simulink model "output_opt_lookup_formation_sim2"  (R2017b)
settings: Solver=VariableStepAuto  StartTime=0.0  StopTime=runtime  RelTol=1e-3
values from neighbouring files (symbols this model uses):
  ess_init_soc = 0.6    [ev_sim_init2.m]
  input_motor_speed = mtr_speed_rad(j)    [output_opt_lookup_formation2.m]
  input_motor_torque = mtr_torque_Nm(i)    [output_opt_lookup_formation2.m]
  K_high = 2    [ev_sim_init2.m]
  K_low = 1    [ev_sim_init2.m]
  TA = torque_allocation(k)    [output_opt_lookup_formation2.m]
undefined symbols (not defined in the file or in its folder): A_frontal, ap00, ap01, ap02, ap03, ap10, ap11, ap12, ap20, ap21, ap30, C_d, ess_cap_scale, ess_fixtemp, ess_max_ah_cap, ess_max_volts, ess_min_volts, ess_module_num, ess_r_chg, ess_r_dis, ess_res_scale_coef, ess_res_scale_fun, ess_soc, ess_tmp, ess_voc, f_rolling, FR, g_gravity, m_map_spd, m_max_trq_IM, m_max_trq_SR, m_min_volts, M_total, p00, p01, p02, p03, p10, p11, p12, p20, p21, p30, R_tire, rho_air
libraries: simulink x3
settings Model: Creator=Robert Wygant  LastModifiedBy=Robert Wygant
settings SolverCC: ZeroCrossControl=DisableAll
settings DebuggingCC: MaxConsecutiveZCsMsg=none

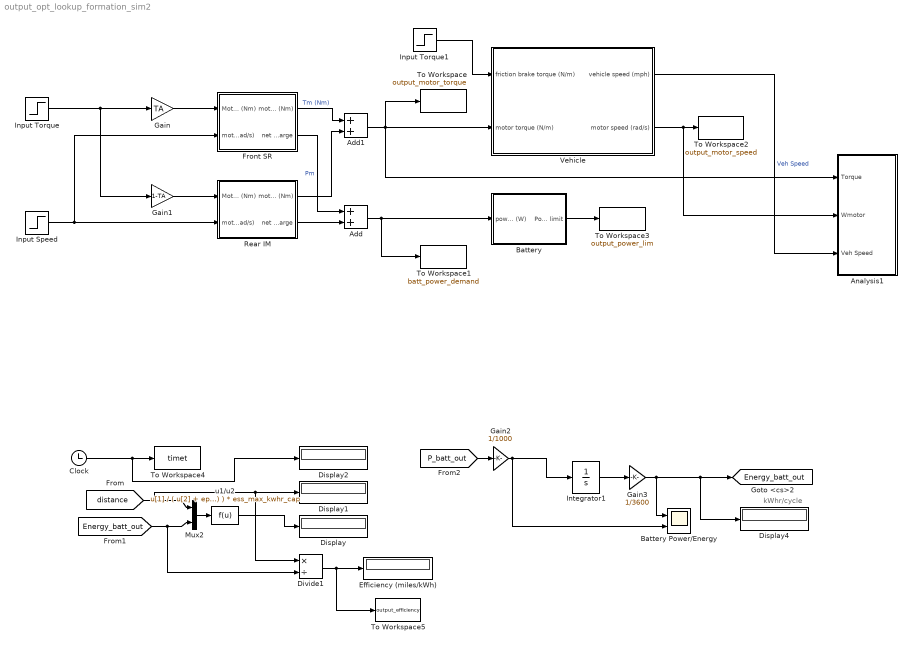
== system output_opt_lookup_formation_sim2 ==
  note: kWhr/cycle
  Add : Sum
  Add1 : Sum
  Analysis1 : Subsystem
  Battery : Subsystem
      mask Display: disp('Battery')
  Battery Power/Energy : Scope  NumInputPorts=2
      settings: Description=Power/Energy
  Clock : Clock
  Display{,1..2,4} (4 alike) : Display
  Divide1 : Product  Inputs=*/
  Efficiency (miles/kWh) : Display
  Front SR : Subsystem
      mask Display: disp('Electric\nMotor')
  Gain : Gain  Gain=TA
  Gain1 : Gain  Gain=1-TA
  Gain2 : Gain  Gain=1/1000  SaturateOnIntegerOverflow=on  OutDataTypeStr=Inherit: Same as input  ParamDataTypeStr=Inherit: Same as input
  Gain3 : Gain  Gain=1/3600  SaturateOnIntegerOverflow=on  OutDataTypeStr=Inherit: Same as input  ParamDataTypeStr=Inherit: Same as input
  Input Speed : Step  Time=0  After=input_motor_speed  SampleTime=0
  Input Torque : Step  Time=0  After=input_motor_torque  SampleTime=0
  Input Torque1 : Step  Time=0.01  After=0  SampleTime=0
  Integrator1 : Integrator  LowerSaturationLimit=0
  Mux2 : Mux  Inputs=2
  Rear IM : Subsystem
      mask Display: disp('Electric\nMotor')
  To Workspace : ToWorkspace  VariableName=output_motor_torque  SampleTime=-1
      settings: Save2DSignal=2-D array (concatenate along first dimension)
  To Workspace1 : ToWorkspace  VariableName=batt_power_demand  SaveFormat=Structure  SampleTime=-1
      settings: Save2DSignal=2-D array (concatenate along first dimension)
  To Workspace2 : ToWorkspace  VariableName=output_motor_speed  SampleTime=-1
      settings: Save2DSignal=2-D array (concatenate along first dimension)
  To Workspace3 : ToWorkspace  VariableName=output_power_lim  SampleTime=-1
      settings: Save2DSignal=2-D array (concatenate along first dimension)
  To Workspace4 : ToWorkspace  VariableName=timet  SampleTime=-1
  To Workspace5 : ToWorkspace  VariableName=output_efficiency  SampleTime=-1
      settings: Save2DSignal=2-D array (concatenate along first dimension)
  Vehicle : Subsystem
      mask Display: disp('Vehicle \nDynamic Model')
  u1/u2 : Fcn  Expr=u[1] / ( u[2] + eps*(u[2] == 0) ) * ess_max_kwhr_cap
  tag scope: Energy_batt_out=global
  wires:
  Front SR/1(motor torque output (Nm)) -> Add1/1  "Tm (Nm)"
  Rear IM/1(motor torque output (Nm)) -> Add1/2
  Add/1 -> Battery/1(power req'd into bus (W)), To Workspace1/1
  Front SR/2(net Power >0 discharge <0 charge) -> Add/1  "Pm"
  Rear IM/2(net Power >0 discharge <0 charge) -> Add/2
  Gain/1 -> Front SR/1(Motor demand Torque (Nm))
  Gain1/1 -> Rear IM/1(Motor demand Torque (Nm))
  Input Torque/1 -> Gain1/1, Gain/1
  Input Speed/1 -> Rear IM/2(motor speed (rad/s)), Front SR/2(motor speed (rad/s))
  Vehicle/1(vehicle speed (mph)) -> Analysis1/3(Veh Speed)  "Veh Speed"
  Add1/1 -> Vehicle/2(motor torque (N/m)), Analysis1/1(Torque), To Workspace/1
  Input Torque1/1 -> Vehicle/1(friction brake torque (N/m))
  Vehicle/2(motor speed (rad/s)) -> Analysis1/2(Wmotor), To Workspace2/1
  Divide1/1 -> To Workspace5/1, Efficiency (miles/kWh)/1
  Gain3/1 -> [Energy_batt_out], Display4/1, Battery Power/Energy/1
  Clock/1 -> To Workspace4/1, Display2/1
  [P_batt_out] -> Gain2/1
  [Energy_batt_out] -> Divide1/2, Mux2/2
  Gain2/1 -> Integrator1/1, Battery Power/Energy/2
  Mux2/1 -> u1/u2/1
  [distance] -> Divide1/1, Display1/1, Mux2/1
  u1/u2/1 -> Display/1
  Integrator1/1 -> Gain3/1
  Battery/1(Power limit) -> To Workspace3/1

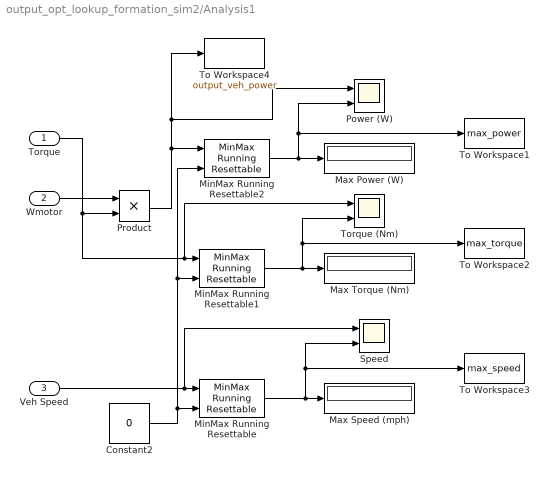
== system output_opt_lookup_formation_sim2/Analysis1 ==
  Torque : Inport
  Wmotor : Inport  Port=2
  Veh Speed : Inport  Port=3
  Constant2 : Constant  Value=0  VectorParams1D=off  SampleTime=-1
  Max Power (W) : Display
  Max Speed (mph) : Display
  Max Torque (Nm) : Display
  MinMax Running Resettable : simulink/Math Operations/MinMax Running Resettable  Function=max  vinit=0.0
  MinMax Running Resettable1 : simulink/Math Operations/MinMax Running Resettable  Function=max  vinit=0.0
  MinMax Running Resettable2 : simulink/Math Operations/MinMax Running Resettable  Function=max  vinit=0.0
  Power (W) : Scope  NumInputPorts=2
  Product : Product
  Speed : Scope  NumInputPorts=2
  To Workspace1 : ToWorkspace  VariableName=max_power  SampleTime=-1
      settings: Save2DSignal=2-D array (concatenate along first dimension)
  To Workspace2 : ToWorkspace  VariableName=max_torque  SampleTime=-1
      settings: Save2DSignal=2-D array (concatenate along first dimension)
  To Workspace3 : ToWorkspace  VariableName=max_speed  SampleTime=-1
      settings: Save2DSignal=2-D array (concatenate along first dimension)
  To Workspace4 : ToWorkspace  VariableName=output_veh_power  SampleTime=-1
      settings: Save2DSignal=2-D array (concatenate along first dimension)
  Torque (Nm) : Scope  NumInputPorts=2
  wires:
  Veh Speed/1 -> Speed/1, MinMax Running Resettable/1
  Wmotor/1 -> Product/1
  Torque/1 -> Torque (Nm)/1, MinMax Running Resettable1/1, Product/2
  Product/1 -> MinMax Running Resettable2/1, To Workspace4/1, Power (W)/1
  Constant2/1 -> MinMax Running Resettable2/2, MinMax Running Resettable1/2, MinMax Running Resettable/2
  MinMax Running Resettable1/1 -> To Workspace2/1, Torque (Nm)/2, Max Torque (Nm)/1
  MinMax Running Resettable/1 -> To Workspace3/1, Speed/2, Max Speed (mph)/1
  MinMax Running Resettable2/1 -> To Workspace1/1, Power (W)/2, Max Power (W)/1

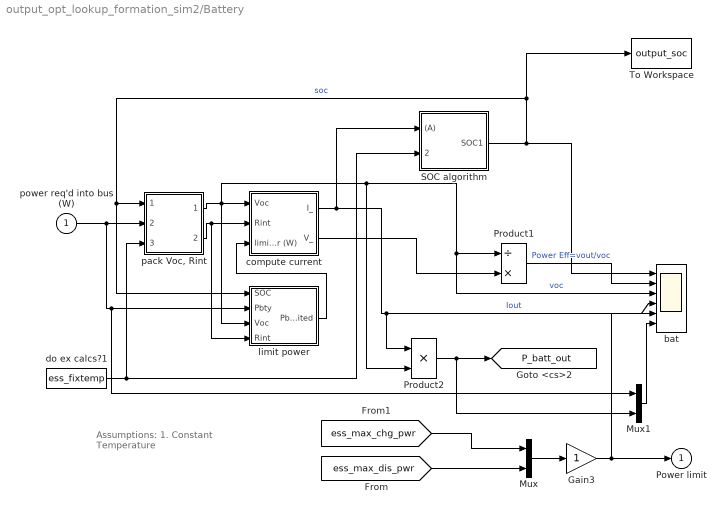
== system output_opt_lookup_formation_sim2/Battery ==
  note: Assumptions:
      | 1. Constant Temperature
  power req'd into bus (W) : Inport
  Gain3 : Gain  SaturateOnIntegerOverflow=on  OutDataTypeStr=Inherit: Same as input  ParamDataTypeStr=Inherit: Same as input
  Mux : Mux  Inputs=2
  Mux1 : Mux  Inputs=2
  Product1 : Product  Inputs=/*  SaturateOnIntegerOverflow=on  InputSameDT=on  OutDataTypeStr=Inherit: Same as first input
  Product2 : Product  Inputs=**  SaturateOnIntegerOverflow=on  InputSameDT=on  OutDataTypeStr=Inherit: Same as first input
  SOC algorithm : Subsystem  AncestorBlock=|
      | lib_energy_storage/Ess Choices/energy
      | storage <ess>/SOC
      | algorithm
      mask Display: disp('SOC\nalgorithm')
  To Workspace : ToWorkspace  VariableName=output_soc  SampleTime=-1
  bat : Scope  NumInputPorts=6
  compute current : Subsystem  AncestorBlock=|
      | lib_energy_storage/Ess Choices/energy
      | storage <ess>/compute
      | current
      mask Display: disp('Compute\nCurrent')
  do ex calcs?1 : Constant  Value=ess_fixtemp
  limit power : Subsystem  AncestorBlock=lib_energy_storage/Ess Choices/energy storage <ess>/limit power
      mask Display: disp('Limit\nPower')
  "pack Voc, Rint" : Subsystem  AncestorBlock=|
      | lib_energy_storage/Ess Choices/energy
      | storage <ess>/pack
      | Voc, Rint
      mask Display: disp('Pack\nVoc,Rint')
  Power limit : Outport  InitialOutput=0
  tag scope: P_batt_out=global
  wires:
  limit power/1("Pbty, limited") -> compute current/3(limited output power (W))
  "pack Voc, Rint"/1(pack open- circuit voltage) -> limit power/3(Voc), compute current/1(Voc), Product1/1, bat/3, Product2/2  "voc"
  "pack Voc, Rint"/2(pack resistance) -> compute current/2(Rint), limit power/4(Rint)
  SOC algorithm/1(SOC1) -> limit power/1(SOC), "pack Voc, Rint"/1(SOC (prev)), To Workspace/1, bat/1  "soc"
  compute current/1(I_) -> SOC algorithm/1((A)), Product2/1, bat/4  "Iout"
  power req'd into bus (W)/1 -> "pack Voc, Rint"/2(req'd battery power (W)), limit power/2(Pbty), Mux1/1
  compute current/2(V_) -> Product1/2
  do ex calcs?1/1 -> "pack Voc, Rint"/3(mod tmp (C)), SOC algorithm/2(tmp (C))
  Mux/1 -> Gain3/1
  Product1/1 -> bat/2  "Power Eff=vout/voc"
  [ess_max_dis_pwr] -> Mux/2
  [ess_max_chg_pwr] -> Mux/1
  Gain3/1 -> Power limit/1, bat/5
  Product2/1 -> [P_batt_out], Mux1/2
  Mux1/1 -> bat/6

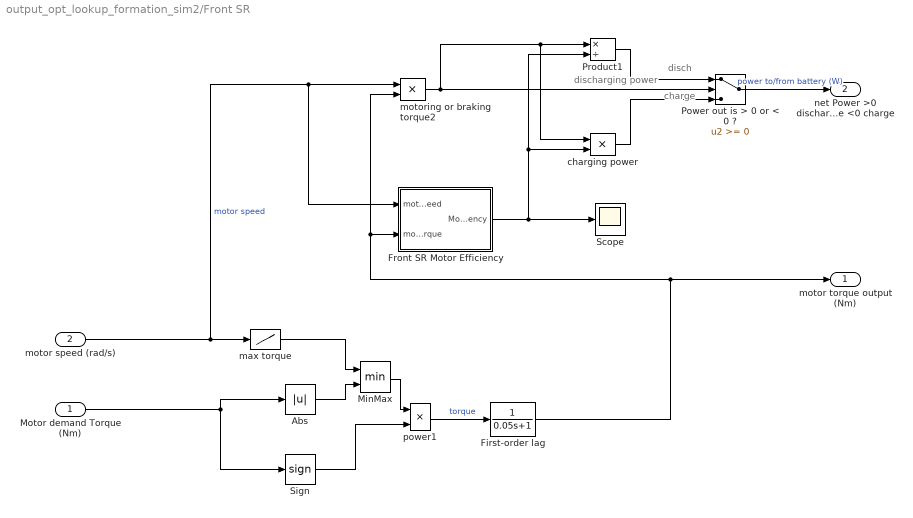
== system output_opt_lookup_formation_sim2/Front SR ==
  note: disch
  note: charge
  note: discharging
      | power
  Motor demand Torque (Nm) : Inport
  motor speed (rad/s) : Inport  Port=2
  Abs : Abs  SaturateOnIntegerOverflow=on
  First-order lag : TransferFcn  Denominator=[0.05 1]
  Front SR Motor Efficiency : Subsystem
      mask Display:
      | color('green')
      | disp("Motor Efficiency")
  MinMax : MinMax  Inputs=2  SaturateOnIntegerOverflow=on  InputSameDT=on
  Power out is > 0 or < 0 ? : Switch  SaturateOnIntegerOverflow=on  InputSameDT=on
  Product1 : Product  Inputs=*/  SaturateOnIntegerOverflow=on  InputSameDT=on  OutDataTypeStr=Inherit: Same as first input
  Scope : Scope
  Sign : Signum
  charging power : Product  SaturateOnIntegerOverflow=on  InputSameDT=on  OutDataTypeStr=Inherit: Same as first input
  max torque : Lookup  InputValues=m_map_spd  Table=m_max_trq_SR  SaturateOnIntegerOverflow=on
  motoring or braking torque2 : Product  SaturateOnIntegerOverflow=on  InputSameDT=on  OutDataTypeStr=Inherit: Same as first input
  power1 : Product  SaturateOnIntegerOverflow=on  InputSameDT=on  OutDataTypeStr=Inherit: Same as first input
  motor torque output (Nm) : Outport  InitialOutput=0
  net Power >0 discharge <0 charge : Outport  Port=2  InitialOutput=0
  wires:
  charging power/1 -> Power out is > 0 or < 0 ?/3
  Product1/1 -> Power out is > 0 or < 0 ?/1
  Power out is > 0 or < 0 ?/1 -> net Power >0 discharge <0 charge/1  "power to/from battery (W)"
  Motor demand Torque (Nm)/1 -> Sign/1, Abs/1
  power1/1 -> First-order lag/1  "torque"
  motoring or braking torque2/1 -> Product1/1, charging power/1, Power out is > 0 or < 0 ?/2
  Abs/1 -> MinMax/2
  MinMax/1 -> power1/1
  Sign/1 -> power1/2
  motor speed (rad/s)/1 -> max torque/1, Front SR Motor Efficiency/1(motor_speed), motoring or braking torque2/1  "motor speed"
  First-order lag/1 -> motor torque output (Nm)/1, Front SR Motor Efficiency/2(motor_torque), motoring or braking torque2/2
  max torque/1 -> MinMax/1
  Front SR Motor Efficiency/1(Motor_efficiency) -> Scope/1, charging power/2, Product1/2

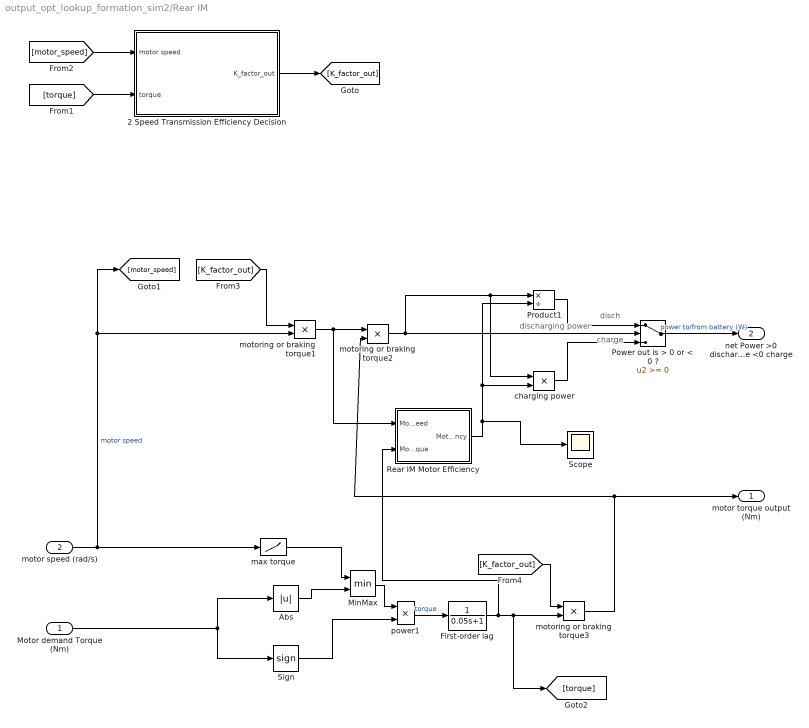
== system output_opt_lookup_formation_sim2/Rear IM ==
  note: disch
  note: charge
  note: discharging
      | power
  Motor demand Torque (Nm) : Inport
  motor speed (rad/s) : Inport  Port=2
  2 Speed Transmission Efficiency Decision : Subsystem
  Abs : Abs  SaturateOnIntegerOverflow=on
  First-order lag : TransferFcn  Denominator=[0.05 1]
  MinMax : MinMax  Inputs=2  SaturateOnIntegerOverflow=on  InputSameDT=on
  Power out is > 0 or < 0 ? : Switch  SaturateOnIntegerOverflow=on  InputSameDT=on
  Product1 : Product  Inputs=*/  SaturateOnIntegerOverflow=on  InputSameDT=on  OutDataTypeStr=Inherit: Same as first input
  Rear IM Motor Efficiency : Subsystem
      mask Display:
      | color('green')
      | disp("Motor Efficiency")
  Scope : Scope
  Sign : Signum
  charging power : Product  SaturateOnIntegerOverflow=on  InputSameDT=on  OutDataTypeStr=Inherit: Same as first input
  max torque : Lookup  InputValues=m_map_spd  Table=m_max_trq_IM  SaturateOnIntegerOverflow=on
  motoring or braking torque1 : Product  SaturateOnIntegerOverflow=on  InputSameDT=on  OutDataTypeStr=Inherit: Same as first input
  motoring or braking torque2 : Product  SaturateOnIntegerOverflow=on  InputSameDT=on  OutDataTypeStr=Inherit: Same as first input
  motoring or braking torque3 : Product  SaturateOnIntegerOverflow=on  InputSameDT=on  OutDataTypeStr=Inherit: Same as first input
  power1 : Product  SaturateOnIntegerOverflow=on  InputSameDT=on  OutDataTypeStr=Inherit: Same as first input
  motor torque output (Nm) : Outport  InitialOutput=0
  net Power >0 discharge <0 charge : Outport  Port=2  InitialOutput=0
  wires:
  charging power/1 -> Power out is > 0 or < 0 ?/3
  Product1/1 -> Power out is > 0 or < 0 ?/1
  Power out is > 0 or < 0 ?/1 -> net Power >0 discharge <0 charge/1  "power to/from battery (W)"
  Motor demand Torque (Nm)/1 -> Abs/1, Sign/1
  power1/1 -> First-order lag/1  "torque"
  motoring or braking torque2/1 -> Product1/1, charging power/1, Power out is > 0 or < 0 ?/2
  Abs/1 -> MinMax/2
  MinMax/1 -> power1/1
  Sign/1 -> power1/2
  max torque/1 -> MinMax/1
  motoring or braking torque1/1 -> Rear IM Motor Efficiency/1(Motor_speed), motoring or braking torque2/1
  motoring or braking torque3/1 -> motoring or braking torque2/2, motor torque output (Nm)/1
  [K_factor_out] -> motoring or braking torque1/1
  [K_factor_out] -> motoring or braking torque3/1
  Rear IM Motor Efficiency/1(Motor_efficiency) -> Scope/1, charging power/2, Product1/2
  [torque] -> 2 Speed Transmission Efficiency Decision/2(torque)
  2 Speed Transmission Efficiency Decision/1(K_factor_out) -> [K_factor_out]
  First-order lag/1 -> Rear IM Motor Efficiency/2(Motor_torque), [torque], motoring or braking torque3/2
  motor speed (rad/s)/1 -> max torque/1, [motor_speed], motoring or braking torque1/2  "motor speed"
  [motor_speed] -> 2 Speed Transmission Efficiency Decision/1(motor speed)

== system output_opt_lookup_formation_sim2/Vehicle ==
  friction brake torque (N/m) : Inport
  motor torque (N/m) : Inport  Port=2
  Dynamics : Subsystem
      mask Display: disp('Vehicle \nDynamic Model')
  Integrator : Integrator  LowerSaturationLimit=0
  m/h --> mps : Gain  Gain=1/3600  SaturateOnIntegerOverflow=on  OutDataTypeStr=Inherit: Same as input  ParamDataTypeStr=Inherit: Same as input
  rad/s --> mph : Gain  Gain=R_tire/1000*0.621371*3600  SaturateOnIntegerOverflow=on  OutDataTypeStr=Inherit: Same as input  ParamDataTypeStr=Inherit: Same as input
  w_r->w_wh : Fcn  Expr=u/FR
  vehicle speed (mph) : Outport
  motor speed (rad/s) : Outport  Port=2
  tag scope: distance=global
  wires:
  motor torque (N/m)/1 -> Dynamics/2(Tm: motor torque (N/m))
  friction brake torque (N/m)/1 -> Dynamics/3("Tfb: friction brake torque (N/m) ")
  w_r->w_wh/1 -> Dynamics/1(wheel speed (rad/s)), rad/s --> mph/1
  rad/s --> mph/1 -> m/h --> mps/1, vehicle speed (mph)/1
  Dynamics/1(motor speed (rad/s)) -> motor speed (rad/s)/1, w_r->w_wh/1
  Integrator/1 -> [distance]
  m/h --> mps/1 -> Integrator/1

== system output_opt_lookup_formation_sim2/Battery/SOC algorithm ==
  note: SOC=(Max Ah capacity-Ah used)/Max Ah capacity
  (A) : Inport
  tmp (C) : Inport  Port=2
  (sec->hrs) : Gain  Gain=1/3600  SaturateOnIntegerOverflow=on  OutDataTypeStr=Inherit: Same as input  ParamDataTypeStr=Inherit: Same as input
  0 <= SOC <= 1 : Saturate  UpperLimit=1  LowerLimit=0
  A-h remaining : Sum  Inputs=-+  SaturateOnIntegerOverflow=on  InputSameDT=on  OutDataTypeStr=Inherit: Same as first input
  Ah used : Integrator  InitialConditionSource=external  InitialCondition=(1-ess_init_soc)*ess_max_ah_cap
  Fcn : Fcn  Expr=1/u
  Fcn1 : Fcn  Expr=(1-ess_init_soc)*u
  SOC : Product  SaturateOnIntegerOverflow=on  InputSameDT=on  OutDataTypeStr=Inherit: Same as first input
  max cap : Lookup  InputValues=ess_tmp  Table=ess_max_ah_cap*ess_cap_scale  SaturateOnIntegerOverflow=on
  SOC1 : Outport  InitialOutput=0
  wires:
  (A)/1 -> (sec->hrs)/1
  (sec->hrs)/1 -> Ah used/1
  Ah used/1 -> A-h remaining/1
  Fcn/1 -> SOC/2
  SOC/1 -> 0 <= SOC <= 1/1
  A-h remaining/1 -> SOC/1
  0 <= SOC <= 1/1 -> SOC1/1
  tmp (C)/1 -> max cap/1
  max cap/1 -> A-h remaining/2, Fcn/1, Fcn1/1
  Fcn1/1 -> Ah used/2

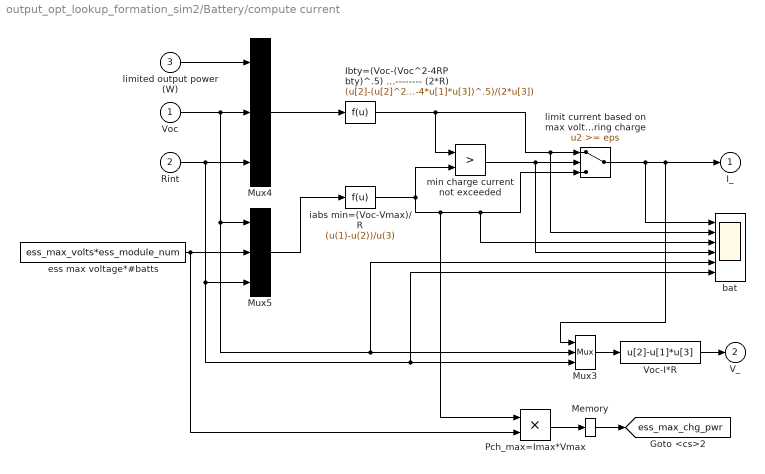
== system output_opt_lookup_formation_sim2/Battery/compute current ==
  Voc : Inport
  Rint : Inport  Port=2
  limited output power (W) : Inport  Port=3
  Ibty=(Voc-(Voc^2-4RPbty)^.5) ----------------------------- (2*R) : Fcn  Expr=(u[2]-(u[2]^2-4*u[1]*u[3])^.5)/(2*u[3])
  Memory : Memory
  Mux3 : Mux  Inputs=3
  Mux4 : Mux  Inputs=3
  Mux5 : Mux  Inputs=3
  Pch_max=Imax*Vmax : Product  SaturateOnIntegerOverflow=on  InputSameDT=on  OutDataTypeStr=Inherit: Same as first input
  Voc-I*R : Fcn  Expr=u[2]-u[1]*u[3]
  bat : Scope  NumInputPorts=6
  ess max voltage*#batts : Constant  Value=ess_max_volts*ess_module_num
  iabs min=(Voc-Vmax)/R : Fcn  Expr=(u(1)-u(2))/u(3)
  limit current based on max voltage during charge : Switch  Threshold=eps  SaturateOnIntegerOverflow=on  InputSameDT=on
  min charge current not exceeded : RelationalOperator  Operator=>  RndMeth=Nearest  InputSameDT=on
  I_ : Outport  InitialOutput=0
  V_ : Outport  Port=2  InitialOutput=0
  tag scope: ess_max_chg_pwr=global
  wires:
  limited output power (W)/1 -> Mux4/1
  Voc/1 -> Mux4/2, Mux5/1, Mux3/2, bat/5
  Rint/1 -> Mux4/3, Mux5/3, Mux3/3, bat/6
  Ibty=(Voc-(Voc^2-4RPbty)^.5) ----------------------------- (2*R)/1 -> min charge current not exceeded/1, limit current based on max voltage during charge/1, bat/2
  iabs min=(Voc-Vmax)/R/1 -> min charge current not exceeded/2, Pch_max=Imax*Vmax/1, limit current based on max voltage during charge/3, bat/3
  limit current based on max voltage during charge/1 -> Mux3/1, I_/1, bat/1
  min charge current not exceeded/1 -> limit current based on max voltage during charge/2, bat/4
  Mux3/1 -> Voc-I*R/1
  Voc-I*R/1 -> V_/1
  Mux4/1 -> Ibty=(Voc-(Voc^2-4RPbty)^.5) ----------------------------- (2*R)/1
  Mux5/1 -> iabs min=(Voc-Vmax)/R/1
  ess max voltage*#batts/1 -> Mux5/2, Pch_max=Imax*Vmax/2
  Pch_max=Imax*Vmax/1 -> Memory/1
  Memory/1 -> [ess_max_chg_pwr]

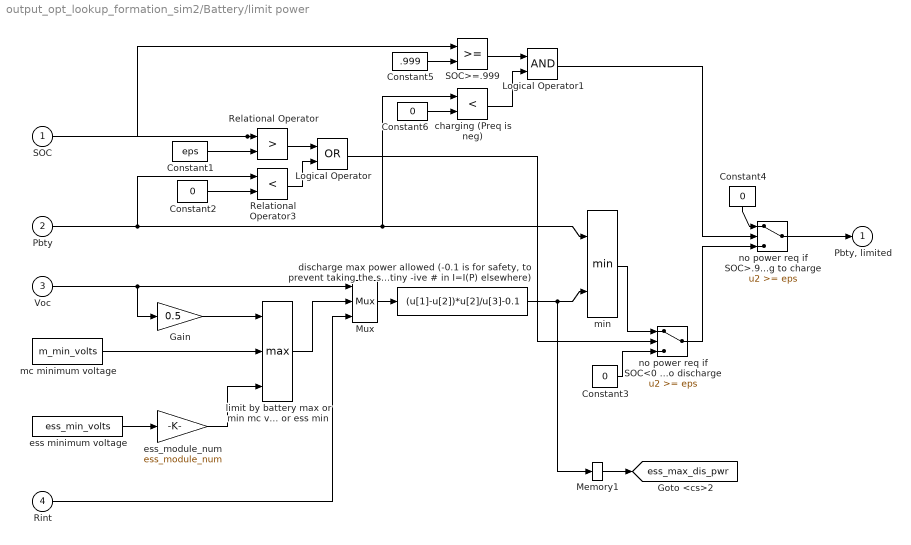
== system output_opt_lookup_formation_sim2/Battery/limit power ==
  SOC : Inport
  Pbty : Inport  Port=2
  Voc : Inport  Port=3
  Rint : Inport  Port=4
  Constant1 : Constant  Value=eps
  Constant{2..4,6} (4 alike) : Constant  Value=0
  Constant5 : Constant  Value=.999
  Gain : Gain  Gain=0.5  SaturateOnIntegerOverflow=on  OutDataTypeStr=Inherit: Same as input  ParamDataTypeStr=Inherit: Same as input
  Logical Operator : Logic  Operator=OR
  Logical Operator1 : Logic
  Memory1 : Memory
  Mux : Mux  Inputs=3
  Relational Operator : RelationalOperator  Operator=>  RndMeth=Nearest  InputSameDT=on
  Relational Operator3 : RelationalOperator  Operator=<  RndMeth=Nearest  InputSameDT=on
  SOC>=.999 : RelationalOperator  RndMeth=Nearest  InputSameDT=on
  charging (Preq is neg) : RelationalOperator  Operator=<  RndMeth=Nearest  InputSameDT=on
  "discharge max power allowed (-0.1 is for safety, to prevent taking the square of a tiny -ive # in I=I(P) elsewhere)" : Fcn  Expr=(u[1]-u[2])*u[2]/u[3]-0.1
  ess minimum voltage : Constant  Value=ess_min_volts
  ess_module_num : Gain  Gain=ess_module_num  SaturateOnIntegerOverflow=on  OutDataTypeStr=Inherit: Same as input  ParamDataTypeStr=Inherit: Same as input
  limit by battery max or min mc voltage or ess min : MinMax  Function=max  Inputs=3  SaturateOnIntegerOverflow=on  InputSameDT=on
  mc minimum voltage : Constant  Value=m_min_volts
  min : MinMax  Inputs=2  SaturateOnIntegerOverflow=on  InputSameDT=on
  no power req if SOC<0 and trying to discharge : Switch  Threshold=eps  SaturateOnIntegerOverflow=on  InputSameDT=on
  no power req if SOC>.999 and trying to charge : Switch  Threshold=eps  SaturateOnIntegerOverflow=on  InputSameDT=on
  "Pbty, limited" : Outport  InitialOutput=0
  tag scope: ess_max_dis_pwr=global
  wires:
  Constant1/1 -> Relational Operator/2
  Relational Operator/1 -> Logical Operator/1
  Pbty/1 -> Relational Operator3/1, charging (Preq is neg)/1, min/1
  Constant2/1 -> Relational Operator3/2
  Relational Operator3/1 -> Logical Operator/2
  Constant3/1 -> no power req if SOC<0 and trying to discharge/3
  Logical Operator/1 -> no power req if SOC<0 and trying to discharge/2
  Voc/1 -> Mux/1, Gain/1
  min/1 -> no power req if SOC<0 and trying to discharge/1
  Mux/1 -> "discharge max power allowed (-0.1 is for safety, to prevent taking the square of a tiny -ive # in I=I(P) elsewhere)"/1
  limit by battery max or min mc voltage or ess min/1 -> Mux/2
  "discharge max power allowed (-0.1 is for safety, to prevent taking the square of a tiny -ive # in I=I(P) elsewhere)"/1 -> min/2, Memory1/1
  mc minimum voltage/1 -> limit by battery max or min mc voltage or ess min/2
  Rint/1 -> Mux/3
  Gain/1 -> limit by battery max or min mc voltage or ess min/1
  ess minimum voltage/1 -> ess_module_num/1
  ess_module_num/1 -> limit by battery max or min mc voltage or ess min/3
  SOC/1 -> Relational Operator/1, SOC>=.999/1
  SOC>=.999/1 -> Logical Operator1/1
  Constant6/1 -> charging (Preq is neg)/2
  charging (Preq is neg)/1 -> Logical Operator1/2
  Constant5/1 -> SOC>=.999/2
  Constant4/1 -> no power req if SOC>.999 and trying to charge/1
  no power req if SOC<0 and trying to discharge/1 -> no power req if SOC>.999 and trying to charge/3
  no power req if SOC>.999 and trying to charge/1 -> "Pbty, limited"/1
  Logical Operator1/1 -> no power req if SOC>.999 and trying to charge/2
  Memory1/1 -> [ess_max_dis_pwr]

== system output_opt_lookup_formation_sim2/Battery/pack Voc, Rint ==
  SOC (prev) : Inport
  req'd battery power (W) : Inport  Port=2
  mod tmp (C) : Inport  Port=3
  #bty : Constant  Value=ess_module_num
  Product : Product  SaturateOnIntegerOverflow=on  InputSameDT=on  OutDataTypeStr=Inherit: Same as first input
  Rchg (ohms) : Subsystem  mask(2-D Table Lookup){xindex=ess_tmp, yindex=ess_soc, table=ess_r_chg}
      mask prompts: xindex "X Index"; yindex "Y Index"
      mask help:
      | Two Dimensional Table Lookup
      | The first input corresponds to X Index and the second input corresponds to the Y Index
      mask init:
      | sftab2chk(xindex,yindex,table);
      mask Help: This block returns a linearly interpolated intersection from the table using the X index (which corresponds to the rows of the table) and the Y index (which corresponds to the columns of the table).  Extrapolation is used.
      mask Display: plot(-10,-10,110,110,[90,50,10],[90,40,30],[90,50,10],[50,26,20],[90,50,10],[22,13,10])
  Rdis (ohms) : Subsystem  mask(2-D Table Lookup){xindex=ess_tmp, yindex=ess_soc, table=ess_r_dis}
      mask prompts: xindex "X Index"; yindex "Y Index"
      mask help:
      | Two Dimensional Table Lookup
      | The first input corresponds to X Index and the second input corresponds to the Y Index
      mask init:
      | sftab2chk(xindex,yindex,table);
      mask Help: This block returns a linearly interpolated intersection from the table using the X index (which corresponds to the rows of the table) and the Y index (which corresponds to the columns of the table).  Extrapolation is used.
      mask Display: plot(-10,-10,110,110,[90,50,10],[90,40,30],[90,50,10],[50,26,20],[90,50,10],[22,13,10])
  Switch : Switch  SaturateOnIntegerOverflow=on  InputSameDT=on
  VOC (V) : Subsystem  mask(2-D Table Lookup){xindex=ess_tmp, yindex=ess_soc, table=ess_voc}
      mask prompts: xindex "X Index"; yindex "Y Index"
      mask help:
      | Two Dimensional Table Lookup
      | The first input corresponds to X Index and the second input corresponds to the Y Index
      mask init:
      | sftab2chk(xindex,yindex,table);
      mask Help: This block returns a linearly interpolated intersection from the table using the X index (which corresponds to the rows of the table) and the Y index (which corresponds to the columns of the table).  Extrapolation is used.
      mask Display: plot(-10,-10,110,110,[90,50,10],[90,40,30],[90,50,10],[50,26,20],[90,50,10],[22,13,10])
  resistance scale fun : Gain  Gain=ess_res_scale_fun(ess_res_scale_coef,ess_module_num,ess_cap_scale)  SaturateOnIntegerOverflow=on  OutDataTypeStr=Inherit: Same as input  ParamDataTypeStr=Inherit: Same as input
  resistance scale fun1 : Gain  Gain=ess_res_scale_fun(ess_res_scale_coef,ess_module_num,ess_cap_scale)  SaturateOnIntegerOverflow=on  OutDataTypeStr=Inherit: Same as input  ParamDataTypeStr=Inherit: Same as input
  pack open- circuit voltage : Outport  InitialOutput=0
  pack resistance : Outport  Port=2  InitialOutput=0
  wires:
  Rchg (ohms)/1(table out) -> resistance scale fun1/1
  Rdis (ohms)/1(table out) -> resistance scale fun/1
  Switch/1 -> pack resistance/1
  #bty/1 -> Product/2
  Product/1 -> pack open- circuit voltage/1
  VOC (V)/1(table out) -> Product/1
  req'd battery power (W)/1 -> Switch/2
  SOC (prev)/1 -> VOC (V)/2(y0), Rdis (ohms)/2(y0), Rchg (ohms)/2(y0)
  mod tmp (C)/1 -> VOC (V)/1(x0), Rdis (ohms)/1(x0), Rchg (ohms)/1(x0)
  resistance scale fun1/1 -> Switch/3
  resistance scale fun/1 -> Switch/1

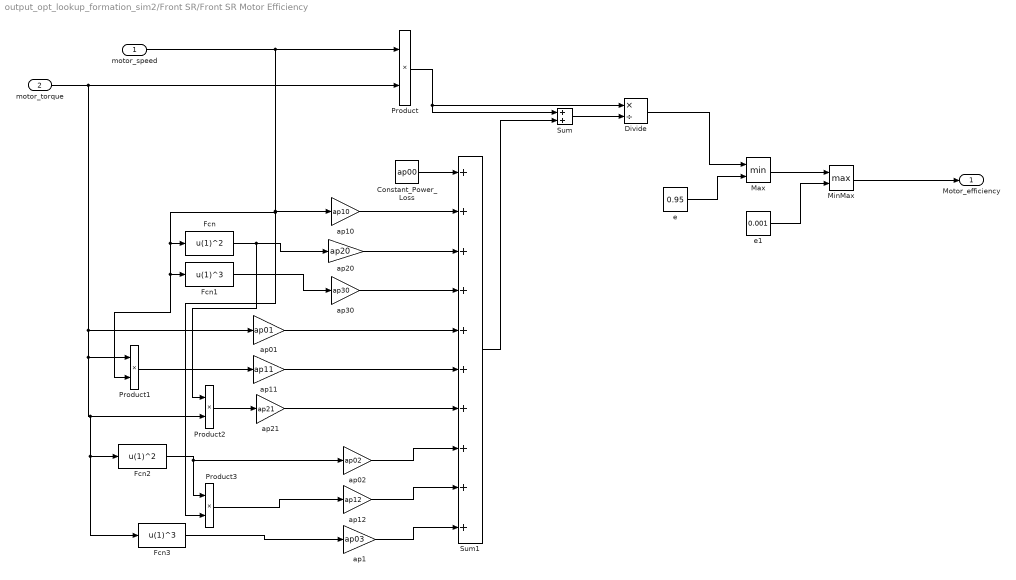
== system output_opt_lookup_formation_sim2/Front SR/Front SR Motor Efficiency ==
  motor_speed : Inport
  motor_torque : Inport  Port=2
  Constant_Power_Loss : Constant  Value=ap00
  Divide : Product  Inputs=*/
  Fcn : Fcn  Expr=u(1)^2
  Fcn1 : Fcn  Expr=u(1)^3
  Fcn2 : Fcn  Expr=u(1)^2
  Fcn3 : Fcn  Expr=u(1)^3
  Max : MinMax  Inputs=2
  MinMax : MinMax  Function=max  Inputs=2
  Product{,1..3} (4 alike) : Product
  Sum : Sum
  Sum1 : Sum  Inputs=++++++++++
  ap01 : Gain  Gain=ap01
  ap02 : Gain  Gain=ap02
  ap1 : Gain  Gain=ap03
  ap10 : Gain  Gain=ap10
  ap11 : Gain  Gain=ap11
  ap12 : Gain  Gain=ap12
  ap20 : Gain  Gain=ap20
  ap21 : Gain  Gain=ap21
  ap30 : Gain  Gain=ap30
  e : Constant  Value=0.95
  e1 : Constant  Value=0.001
  Motor_efficiency : Outport
  wires:
  e/1 -> Max/2
  Fcn3/1 -> ap1/1
  ap1/1 -> Sum1/10
  ap12/1 -> Sum1/9
  Product3/1 -> ap12/1
  motor_torque/1 -> Product/2, Product1/1, Product2/2, Fcn2/1, Fcn3/1, ap01/1
  ap01/1 -> Sum1/5
  ap11/1 -> Sum1/6
  ap21/1 -> Sum1/7
  ap02/1 -> Sum1/8
  Fcn2/1 -> ap02/1, Product3/1
  Product2/1 -> ap21/1
  Product1/1 -> ap11/1
  ap30/1 -> Sum1/4
  Fcn1/1 -> ap30/1
  Fcn/1 -> ap20/1, Product2/1
  ap20/1 -> Sum1/3
  ap10/1 -> Sum1/2
  Constant_Power_Loss/1 -> Sum1/1
  motor_speed/1 -> Product/1, Product3/2, Fcn/1, Fcn1/1, Product1/2, ap10/1
  Divide/1 -> Max/1
  Sum1/1 -> Sum/2
  Sum/1 -> Divide/2
  Product/1 -> Divide/1, Sum/1
  Max/1 -> MinMax/1
  e1/1 -> MinMax/2
  MinMax/1 -> Motor_efficiency/1

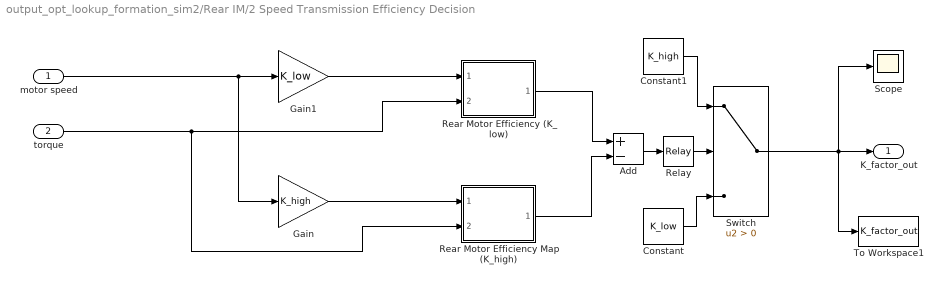
== system output_opt_lookup_formation_sim2/Rear IM/2 Speed Transmission Efficiency Decision ==
  motor speed : Inport
  torque : Inport  Port=2
  Add : Sum  Inputs=+-
  Constant : Constant  Value=K_low
  Constant1 : Constant  Value=K_high
  Gain : Gain  Gain=K_high
  Gain1 : Gain  Gain=K_low
  Rear Motor Efficiency (K_low) : Subsystem
      mask Display:
      | color('green')
      | disp("Motor Efficiency")
  Rear Motor Efficiency Map (K_high) : Subsystem
      mask Display:
      | color('green')
      | disp("Motor Efficiency")
  Relay : Relay  OnSwitchValue=0.15  OffSwitchValue=-.15  OffOutputValue=-1
  Scope : Scope
  Switch : Switch  Criteria=u2 > Threshold
  To Workspace1 : ToWorkspace  VariableName=K_factor_out  SampleTime=-1
      settings: Save2DSignal=2-D array (concatenate along first dimension)
  K_factor_out : Outport
  wires:
  Constant1/1 -> Switch/1
  Constant/1 -> Switch/3
  Add/1 -> Relay/1
  torque/1 -> Rear Motor Efficiency Map (K_high)/2(Motor_torque), Rear Motor Efficiency (K_low)/2(Motor_torque)
  Rear Motor Efficiency (K_low)/1(Motor_efficiency) -> Add/1
  Rear Motor Efficiency Map (K_high)/1(Motor_efficiency) -> Add/2
  Gain1/1 -> Rear Motor Efficiency (K_low)/1(Motor_speed)
  Gain/1 -> Rear Motor Efficiency Map (K_high)/1(Motor_speed)
  motor speed/1 -> Gain/1, Gain1/1
  Switch/1 -> To Workspace1/1, Scope/1, K_factor_out/1
  Relay/1 -> Switch/2

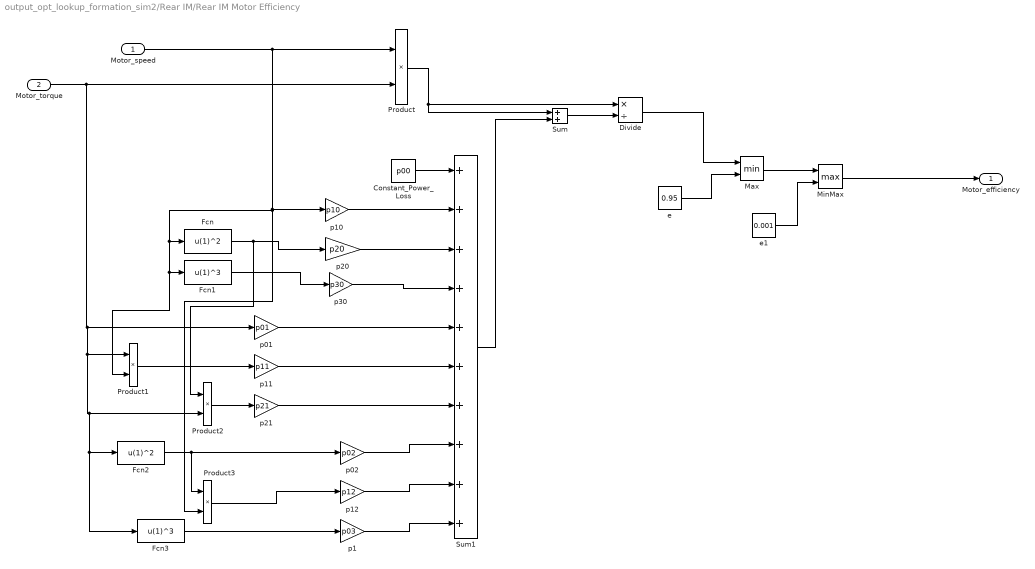
== system output_opt_lookup_formation_sim2/Rear IM/Rear IM Motor Efficiency ==
  Motor_speed : Inport
  Motor_torque : Inport  Port=2
  Constant_Power_Loss : Constant  Value=p00
  Divide : Product  Inputs=*/
  Fcn : Fcn  Expr=u(1)^2
  Fcn1 : Fcn  Expr=u(1)^3
  Fcn2 : Fcn  Expr=u(1)^2
  Fcn3 : Fcn  Expr=u(1)^3
  Max : MinMax  Inputs=2
  MinMax : MinMax  Function=max  Inputs=2
  Product{,1..3} (4 alike) : Product
  Sum : Sum
  Sum1 : Sum  Inputs=++++++++++
  e : Constant  Value=0.95
  e1 : Constant  Value=0.001
  p01 : Gain  Gain=p01
  p02 : Gain  Gain=p02
  p1 : Gain  Gain=p03
  p10 : Gain  Gain=p10
  p11 : Gain  Gain=p11
  p12 : Gain  Gain=p12
  p20 : Gain  Gain=p20
  p21 : Gain  Gain=p21
  p30 : Gain  Gain=p30
  Motor_efficiency : Outport
  wires:
  Max/1 -> MinMax/1
  e/1 -> Max/2
  Fcn3/1 -> p1/1
  p1/1 -> Sum1/10
  p12/1 -> Sum1/9
  Product3/1 -> p12/1
  Motor_torque/1 -> Product/2, p01/1, Product1/1, Product2/2, Fcn2/1, Fcn3/1
  p01/1 -> Sum1/5
  p11/1 -> Sum1/6
  p21/1 -> Sum1/7
  p02/1 -> Sum1/8
  Fcn2/1 -> p02/1, Product3/1
  Product2/1 -> p21/1
  Product1/1 -> p11/1
  p30/1 -> Sum1/4
  Fcn1/1 -> p30/1
  Fcn/1 -> p20/1, Product2/1
  p20/1 -> Sum1/3
  p10/1 -> Sum1/2
  Constant_Power_Loss/1 -> Sum1/1
  Motor_speed/1 -> Product/1, p10/1, Fcn/1, Fcn1/1, Product1/2, Product3/2
  Divide/1 -> Max/1
  Sum1/1 -> Sum/2
  Sum/1 -> Divide/2
  Product/1 -> Divide/1, Sum/1
  e1/1 -> MinMax/2
  MinMax/1 -> Motor_efficiency/1

== system output_opt_lookup_formation_sim2/Vehicle/Dynamics ==
  note: Assumptions:
      | 1. No loss
      | 2. Small pinion gear inertia
      | 3. Longitudinal dynamics only
  wheel speed (rad/s) : Inport
  Tm: motor torque (N/m) : Inport  Port=2
  "Tfb: friction brake torque (N/m) " : Inport  Port=3
  Aero Drag : Fcn  Expr=0.5*A_frontal*rho_air* C_d*u^2*R_tire^3/FR^2
  Constant : Constant
  Constant1 : Constant  Value=0
  Gain : Gain  Gain=FR  SaturateOnIntegerOverflow=on  OutDataTypeStr=Inherit: Same as input  ParamDataTypeStr=Inherit: Same as input
  Integrator1 : Integrator  InitialCondition=0.1  LimitOutput=on  LowerSaturationLimit=0.1
  Rolling Resistance : Fcn  Expr=M_total*g_gravity*f_rolling*R_tire*u
  Sum : Sum  Inputs=+---  SaturateOnIntegerOverflow=on
  Switch : Switch  Threshold=0.001  SaturateOnIntegerOverflow=on
  To Workspace3 : ToWorkspace  VariableName=T_fb  SampleTime=-1
  Vehicle Propulsion : Fcn  Expr=u/(M_total*R_tire^2/FR)
  motor speed (rad/s) : Outport  InitialOutput=0
  wires:
  Vehicle Propulsion/1 -> Integrator1/1
  Integrator1/1 -> motor speed (rad/s)/1, Aero Drag/1
  Rolling Resistance/1 -> Sum/3  "Roll Resis"
  Aero Drag/1 -> Sum/4
  wheel speed (rad/s)/1 -> Switch/2
  Tm: motor torque (N/m)/1 -> Gain/1  "Tm"
  Constant1/1 -> Switch/3
  Constant/1 -> Switch/1
  Switch/1 -> Rolling Resistance/1
  Gain/1 -> Sum/1
  "Tfb: friction brake torque (N/m) "/1 -> Sum/2, To Workspace3/1  "Tf"
  Sum/1 -> Vehicle Propulsion/1

== system output_opt_lookup_formation_sim2/Battery/pack Voc, Rint/Rchg (ohms) ==
  x0 : Inport
  y0 : Inport  Port=2
  Mux : Mux  Inputs=2
  S-function : S-Function  FunctionName=sftable2  Parameters=xindex, yindex, table  SFunctionDeploymentMode=off  EnableBusSupport=off
  table out : Outport  InitialOutput=0
  wires:
  y0/1 -> Mux/2
  S-function/1 -> table out/1
  x0/1 -> Mux/1
  Mux/1 -> S-function/1

== system output_opt_lookup_formation_sim2/Battery/pack Voc, Rint/Rdis (ohms) ==
  x0 : Inport
  y0 : Inport  Port=2
  Mux : Mux  Inputs=2
  S-function : S-Function  FunctionName=sftable2  Parameters=xindex, yindex, table  SFunctionDeploymentMode=off  EnableBusSupport=off
  table out : Outport  InitialOutput=0
  wires:
  y0/1 -> Mux/2
  S-function/1 -> table out/1
  x0/1 -> Mux/1
  Mux/1 -> S-function/1

== system output_opt_lookup_formation_sim2/Battery/pack Voc, Rint/VOC (V) ==
  x0 : Inport
  y0 : Inport  Port=2
  Mux : Mux  Inputs=2
  S-function : S-Function  FunctionName=sftable2  Parameters=xindex, yindex, table  SFunctionDeploymentMode=off  EnableBusSupport=off
  table out : Outport  InitialOutput=0
  wires:
  y0/1 -> Mux/2
  S-function/1 -> table out/1
  x0/1 -> Mux/1
  Mux/1 -> S-function/1

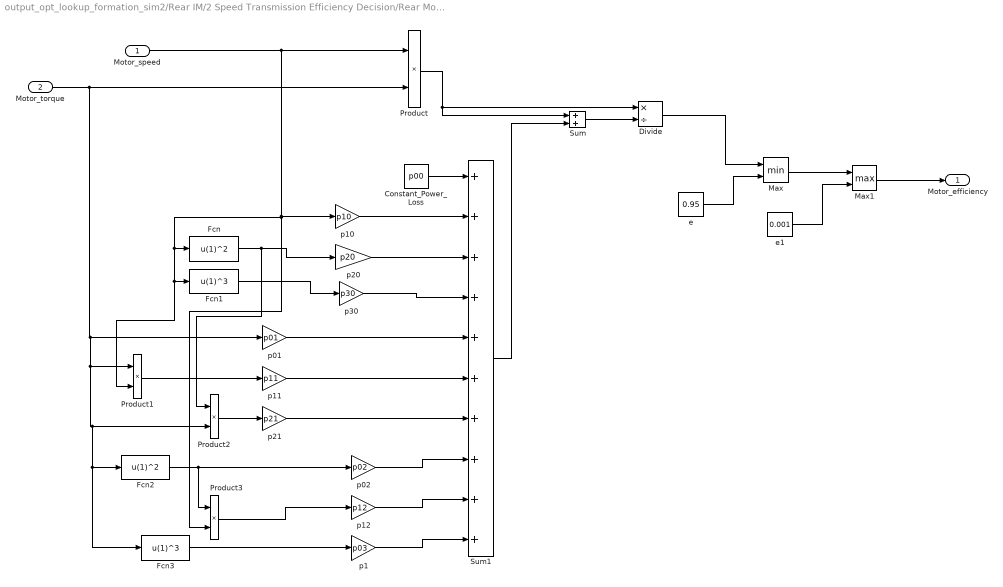
== system output_opt_lookup_formation_sim2/Rear IM/2 Speed Transmission Efficiency Decision/Rear Motor Efficiency (K_low) ==
  Motor_speed : Inport
  Motor_torque : Inport  Port=2
  Constant_Power_Loss : Constant  Value=p00
  Divide : Product  Inputs=*/
  Fcn : Fcn  Expr=u(1)^2
  Fcn1 : Fcn  Expr=u(1)^3
  Fcn2 : Fcn  Expr=u(1)^2
  Fcn3 : Fcn  Expr=u(1)^3
  Max : MinMax  Inputs=2
  Max1 : MinMax  Function=max  Inputs=2
  Product{,1..3} (4 alike) : Product
  Sum : Sum
  Sum1 : Sum  Inputs=++++++++++
  e : Constant  Value=0.95
  e1 : Constant  Value=0.001
  p01 : Gain  Gain=p01
  p02 : Gain  Gain=p02
  p1 : Gain  Gain=p03
  p10 : Gain  Gain=p10
  p11 : Gain  Gain=p11
  p12 : Gain  Gain=p12
  p20 : Gain  Gain=p20
  p21 : Gain  Gain=p21
  p30 : Gain  Gain=p30
  Motor_efficiency : Outport
  wires:
  e/1 -> Max/2
  Fcn3/1 -> p1/1
  p1/1 -> Sum1/10
  p12/1 -> Sum1/9
  Product3/1 -> p12/1
  Motor_torque/1 -> Product/2, p01/1, Product1/1, Product2/2, Fcn2/1, Fcn3/1
  p01/1 -> Sum1/5
  p11/1 -> Sum1/6
  p21/1 -> Sum1/7
  p02/1 -> Sum1/8
  Fcn2/1 -> p02/1, Product3/1
  Product2/1 -> p21/1
  Product1/1 -> p11/1
  p30/1 -> Sum1/4
  Fcn1/1 -> p30/1
  Fcn/1 -> p20/1, Product2/1
  p20/1 -> Sum1/3
  p10/1 -> Sum1/2
  Constant_Power_Loss/1 -> Sum1/1
  Motor_speed/1 -> Product/1, p10/1, Fcn/1, Fcn1/1, Product1/2, Product3/2
  Divide/1 -> Max/1
  Sum1/1 -> Sum/2
  Sum/1 -> Divide/2
  Product/1 -> Divide/1, Sum/1
  Max/1 -> Max1/1
  Max1/1 -> Motor_efficiency/1
  e1/1 -> Max1/2

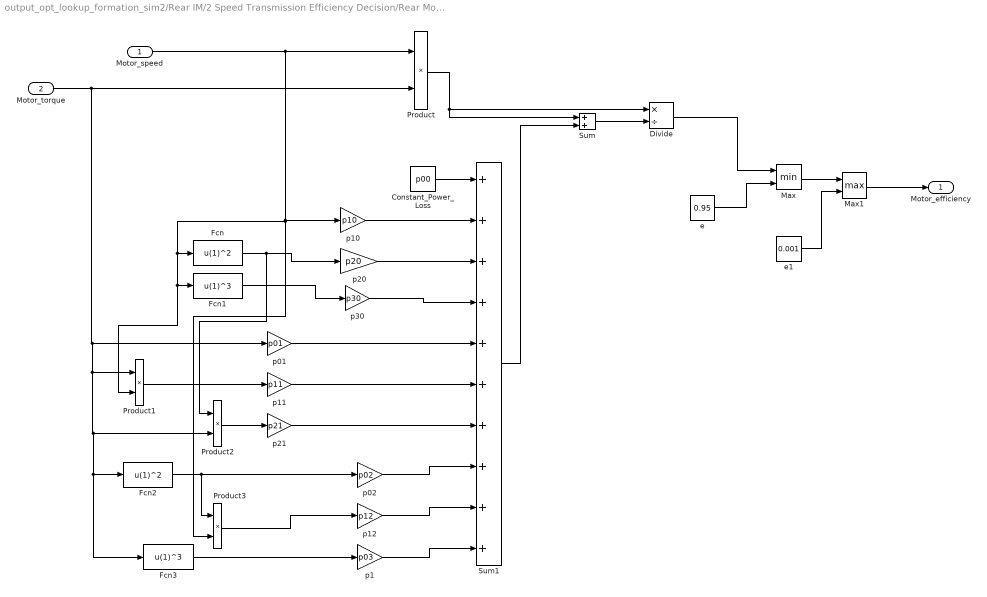
== system output_opt_lookup_formation_sim2/Rear IM/2 Speed Transmission Efficiency Decision/Rear Motor Efficiency Map (K_high) ==
  Motor_speed : Inport
  Motor_torque : Inport  Port=2
  Constant_Power_Loss : Constant  Value=p00
  Divide : Product  Inputs=*/
  Fcn : Fcn  Expr=u(1)^2
  Fcn1 : Fcn  Expr=u(1)^3
  Fcn2 : Fcn  Expr=u(1)^2
  Fcn3 : Fcn  Expr=u(1)^3
  Max : MinMax  Inputs=2
  Max1 : MinMax  Function=max  Inputs=2
  Product{,1..3} (4 alike) : Product
  Sum : Sum
  Sum1 : Sum  Inputs=++++++++++
  e : Constant  Value=0.95
  e1 : Constant  Value=0.001
  p01 : Gain  Gain=p01
  p02 : Gain  Gain=p02
  p1 : Gain  Gain=p03
  p10 : Gain  Gain=p10
  p11 : Gain  Gain=p11
  p12 : Gain  Gain=p12
  p20 : Gain  Gain=p20
  p21 : Gain  Gain=p21
  p30 : Gain  Gain=p30
  Motor_efficiency : Outport
  wires:
  e/1 -> Max/2
  Fcn3/1 -> p1/1
  p1/1 -> Sum1/10
  p12/1 -> Sum1/9
  Product3/1 -> p12/1
  Motor_torque/1 -> Product/2, p01/1, Product1/1, Product2/2, Fcn2/1, Fcn3/1
  p01/1 -> Sum1/5
  p11/1 -> Sum1/6
  p21/1 -> Sum1/7
  p02/1 -> Sum1/8
  Fcn2/1 -> p02/1, Product3/1
  Product2/1 -> p21/1
  Product1/1 -> p11/1
  p30/1 -> Sum1/4
  Fcn1/1 -> p30/1
  Fcn/1 -> p20/1, Product2/1
  p20/1 -> Sum1/3
  p10/1 -> Sum1/2
  Constant_Power_Loss/1 -> Sum1/1
  Motor_speed/1 -> Product/1, p10/1, Fcn/1, Fcn1/1, Product1/2, Product3/2
  Divide/1 -> Max/1
  Sum1/1 -> Sum/2
  Sum/1 -> Divide/2
  Product/1 -> Divide/1, Sum/1
  Max/1 -> Max1/1
  Max1/1 -> Motor_efficiency/1
  e1/1 -> Max1/2
